simulink model "HEVP0"  (R2026b)
settings: Solver=VariableStepAuto
undefined symbols (not defined in the file): Diff, Eng, Lock, PlntDiffrntlP0Ratio, PlntDriveshftDamp, PlntDriveshftStiff, PlntTransEffTempBpt, PlntTransGearRatioVect, Trans, up
libraries: autolibsharedcoupling x2, autolibsharedtransfixedgear x1, autolibtrqconv x1, autolibpowerinfoutils x1
settings Model: ModifiedByFormat=The MathWorks, Inc.  Creator=The MathWorks, Inc.  LastModifiedBy=The MathWorks, Inc.
settings RTWCC: DLArmComputeVersion=19.05

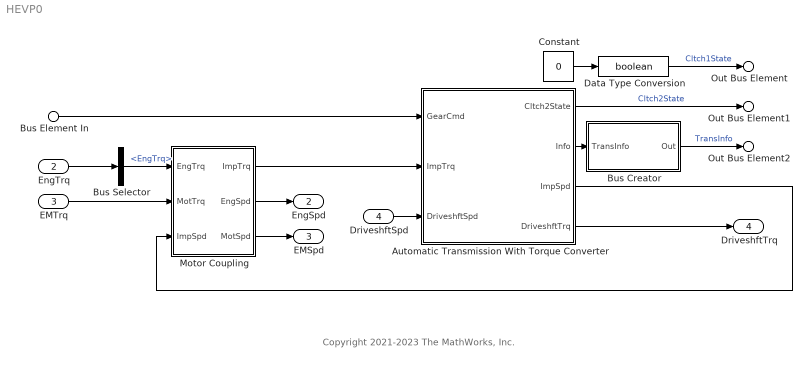
== system HEVP0 ==
  note: Copyright 2021-2023 The MathWorks, Inc.
  Bus Element In : Inport  PortName=Cntrl  Element=Trans.GearCmd
  EngTrq : Inport  Port=2
  EMTrq : Inport  Port=3
  DriveshftSpd : Inport  Port=4
  Automatic Transmission With Torque Converter : Subsystem  VariantControl=1
  Bus Selector : BusSelector  OutputSignals=EngTrq
  Bus Creator : Subsystem
  Constant : Constant  Value=0  SampleTime=-1
  Data Type Conversion : DataTypeConversion  OutDataTypeStr=boolean  SaturateOnIntegerOverflow=off  RndMeth=Floor
  Motor Coupling : Subsystem
  Out Bus Element : Outport  PortName=TransInfo  Element=Cltch1State
  Out Bus Element1 : Outport  PortName=TransInfo  Element=Cltch2State
  Out Bus Element2 : Outport  PortName=TransInfo  Element=Info
  EngSpd : Outport  Port=2  VectorParamsAs1DForOutWhenUnconnected=off  BusOutputAsStruct=on
  EMSpd : Outport  Port=3  VectorParamsAs1DForOutWhenUnconnected=off  BusOutputAsStruct=on
  DriveshftTrq : Outport  Port=4  VectorParamsAs1DForOutWhenUnconnected=off
  wires:
  Automatic Transmission With Torque Converter/4(DriveshftTrq) -> DriveshftTrq/1
  DriveshftSpd/1 -> Automatic Transmission With Torque Converter/3(DriveshftSpd)
  Motor Coupling/2(EngSpd) -> EngSpd/1
  Motor Coupling/3(MotSpd) -> EMSpd/1
  EngTrq/1 -> Bus Selector/1
  EMTrq/1 -> Motor Coupling/2(MotTrq)
  Motor Coupling/1(ImpTrq) -> Automatic Transmission With Torque Converter/2(ImpTrq)
  Bus Element In/1 -> Automatic Transmission With Torque Converter/1(GearCmd)
  Automatic Transmission With Torque Converter/3(ImpSpd) -> Motor Coupling/3(ImpSpd)
  Data Type Conversion/1 -> Out Bus Element/1  "Cltch1State"
  Automatic Transmission With Torque Converter/1(Cltch2State) -> Out Bus Element1/1  "Cltch2State"
  Constant/1 -> Data Type Conversion/1
  Bus Creator/1(Out) -> Out Bus Element2/1  "TransInfo"
  Bus Selector/1 -> Motor Coupling/1(EngTrq)  "<EngTrq>"
  Automatic Transmission With Torque Converter/2(Info) -> Bus Creator/1(TransInfo)

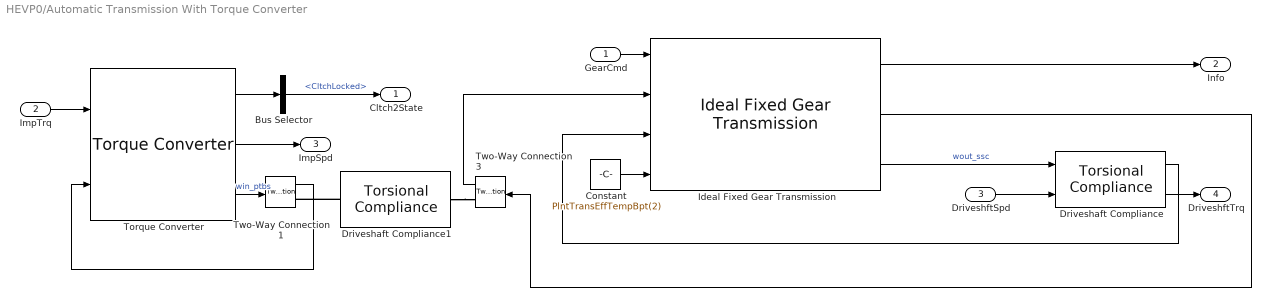
== system HEVP0/Automatic Transmission With Torque Converter ==
  GearCmd : Inport
  ImpTrq : Inport  Port=2
  DriveshftSpd : Inport  Port=3
  Bus Selector : BusSelector  OutputSignals=Cltch.CltchLocked
  Constant : Constant  Value=PlntTransEffTempBpt(2)  SampleTime=-1
  Driveshaft Compliance : autolibsharedcoupling/Torsional Compliance  port_config=Simulink  extInfo=off  k=PlntDriveshftStiff  b=PlntDriveshftDamp  theta_o=PlntDriveshftInitDeflect  domega_o=PlntDriveshftInitVel  omega_c=PlntDriveshftDampCutoffFreq  blkID=0  aMode=1
  Driveshaft Compliance1 : autolibsharedcoupling/Torsional Compliance  port_config=Two-way connection  extInfo=off  k=PlntDriveshftStiff  b=PlntDriveshftDamp  theta_o=PlntDriveshftInitDeflect  domega_o=PlntDriveshftInitVel  omega_c=PlntDriveshftDampCutoffFreq  blkID=0  aMode=1
  Ideal Fixed Gear Transmission : autolibsharedtransfixedgear/Ideal Fixed Gear Transmission  VariantControl=0  TransEffModelPopup=Gear, input torque, input speed, and temperature  gearInterp=Linear point-slope  TrqCnvrtrType=None  G=PlntTransGearNumVect  Trq_bpts=PlntTransEffTrqBpt  omega_bpts=PlntTransEffSpdBpt  Temp_bpts=PlntTransEffTempBpt  N=PlntTransGearRatioVect  Jout=PlntTransInertiaVect  bout=PlntTransDampVect  eta=PlntTransEffVect  eta_tbl=PlntTransEffTbl  G_o=PlntTransInitGear  omega_o=PlntTransInitOutVel  omegaN_o=PlntTransInitNtrlInVel  tau_s=PlntTransShftTimeCnst  phi=[ 0 0.50 0.60 0.70 0.80 0.87 0.92 0.94 0.96 0.97]  psi=[12.2938 12.8588 13.1452 13.6285 14.6163 16.2675 19.3503 22.1046 29.9986 50.00]  zeta=[ 2.2320 1.5462 1.4058 1.2746 1.1528 1.0732 1.0192 0.9983 0.9983 0.9983]  philu=0.96  omegau=0  omegal=0  tauTC=0.1  maxAbsSpd=5e3  aMode=6
  Torque Converter : autolibtrqconv/Torque Converter  TCType=Lock-up  port_config=Simulink  Ji=PlntTrqConvrtrImpInertia  bi=PlntTrqConvrtrImpDamp  Jt=PlntTrqConvrtrTurbInertia  bt=PlntTrqConvrtrTurbDamp  omegai_o=PlntTrqConvrtrImpInitVel  omegat_o=PlntTrqConvrtrTurbInitVel  phi=PlntTrqConvrtrSpdRatioVect  KType=Input speed / sqrt(input torque)  psi=PlntTrqConvrtrCapVect  zeta=PlntTrqConvrtrTrqRatioVect  tauTC=PlntTrqConvrtrTimeCnst  InterpMethod=Linear  Reff=PlntTrqConvrtrCltchRadius  mus=PlntTrqConvrtrCltchStatFric  muk=PlntTrqConvrtrCltchKinFric  ClutchLocked=off  philu=PlntTrqConvrtrCltchLckUpSpdRatio  omegal=PlntTrqConvrtrCltchMinLckUpEngdSpd  omegau=PlntTrqConvrtrCltchMinLckUpDisengdSpd  K_c=PlntTrqConvrtrCltchLckUpForceGain  tauC=PlntTrqConvrtrCltchLckUpTimeCnst  maxAbsSpd=5e3  tau_dl=3000
      settings: AttributesFormatString="Lock-up type:  %<TCType>"
  Two-Way Connection1 : TwoWayConnection
  Two-Way Connection3 : TwoWayConnection
  Cltch2State : Outport  VectorParamsAs1DForOutWhenUnconnected=off
  Info : Outport  Port=2  VectorParamsAs1DForOutWhenUnconnected=off
  ImpSpd : Outport  Port=3  VectorParamsAs1DForOutWhenUnconnected=off
  DriveshftTrq : Outport  Port=4  VectorParamsAs1DForOutWhenUnconnected=off
  wires:
  DriveshftSpd/1 -> Driveshaft Compliance/2
  Torque Converter/3 -> Two-Way Connection1/1  "win_ptbs"
  Two-Way Connection3/1 -> Ideal Fixed Gear Transmission/2
  Torque Converter/2 -> ImpSpd/1
  ImpTrq/1 -> Torque Converter/1
  GearCmd/1 -> Ideal Fixed Gear Transmission/1
  Ideal Fixed Gear Transmission/1 -> Info/1
  Torque Converter/1 -> Bus Selector/1
  Ideal Fixed Gear Transmission/2 -> Two-Way Connection3/1
  Driveshaft Compliance/1 -> Ideal Fixed Gear Transmission/3
  Two-Way Connection1/1 -> Torque Converter/2
  Ideal Fixed Gear Transmission/3 -> Driveshaft Compliance/1  "wout_ssc"
  Bus Selector/1 -> Cltch2State/1  "<CltchLocked>"
  Constant/1 -> Ideal Fixed Gear Transmission/4
  Driveshaft Compliance/2 -> DriveshftTrq/1
  connections:
  Driveshaft Compliance1/RConn1 -- Two-Way Connection3/RConn1
  Driveshaft Compliance1/LConn1 -- Two-Way Connection1/RConn1

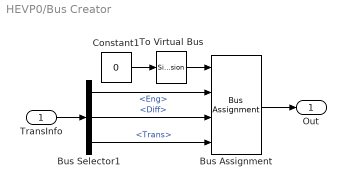
== system HEVP0/Bus Creator ==
  TransInfo : Inport
  Bus Assignment : BusAssignment  AssignedSignals=Eng,Diff,Trans
  Bus Selector1 : BusSelector  OutputSignals=Eng,Diff,Trans
  Constant1 : Constant  Value=0  OutDataTypeStr=Bus: InfoBUS  SampleTime=Inf
  To Virtual Bus : SignalConversion  ConversionOutput=Virtual bus  OverrideOpt=off
  Out : Outport
  wires:
  To Virtual Bus/1 -> Bus Assignment/1
  Constant1/1 -> To Virtual Bus/1
  TransInfo/1 -> Bus Selector1/1
  Bus Selector1/3 -> Bus Assignment/4  "<Trans>"
  Bus Selector1/1 -> Bus Assignment/2  "<Eng>"
  Bus Selector1/2 -> Bus Assignment/3  "<Diff>"
  Bus Assignment/1 -> Out/1

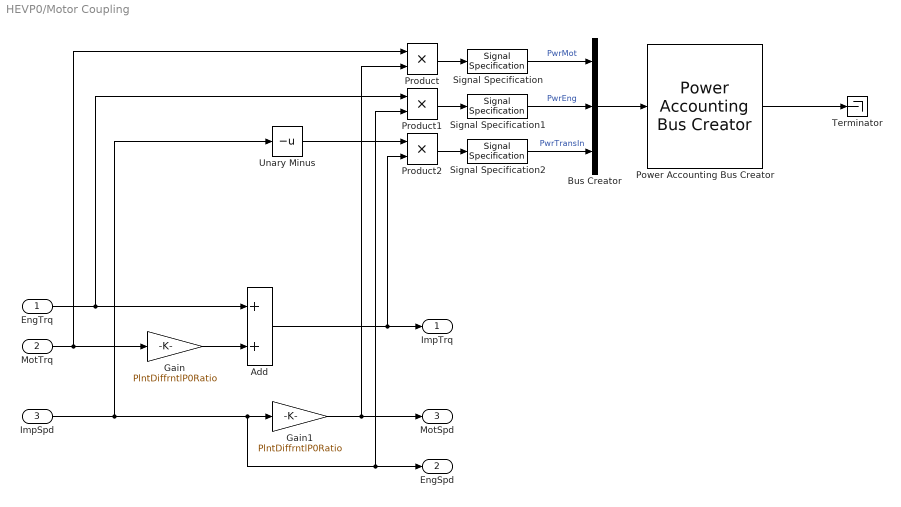
== system HEVP0/Motor Coupling ==
  EngTrq : Inport
  MotTrq : Inport  Port=2
  ImpSpd : Inport  Port=3
  Add : Sum
  Bus Creator : BusCreator  Inputs=3
  Gain : Gain  Gain=PlntDiffrntlP0Ratio
  Gain1 : Gain  Gain=PlntDiffrntlP0Ratio
  Power Accounting Bus Creator : autolibpowerinfoutils/Power Accounting Bus Creator  AssctBlkSelPopup=Parent  RefBlkName='libraryname/blkname'  PwrTrnsfrdCheckBox=on  PwrNotTrnsfrdCheckBox=off  PwrStoredCheckBox=off  aMode=aMode
  Product : Product
  Product1 : Product
  Product2 : Product
  Signal Specification : SignalSpecification  Unit=W
  Signal Specification1 : SignalSpecification  Unit=W
  Signal Specification2 : SignalSpecification  Unit=W
  Terminator : Terminator
  Unary Minus : UnaryMinus
  ImpTrq : Outport  VectorParamsAs1DForOutWhenUnconnected=off
  EngSpd : Outport  Port=2  VectorParamsAs1DForOutWhenUnconnected=off  BusOutputAsStruct=on
  MotSpd : Outport  Port=3  VectorParamsAs1DForOutWhenUnconnected=off  BusOutputAsStruct=on
  wires:
  Unary Minus/1 -> Product2/1
  Product2/1 -> Signal Specification2/1
  Product1/1 -> Signal Specification1/1
  Product/1 -> Signal Specification/1
  Signal Specification1/1 -> Bus Creator/2  "PwrEng"
  Power Accounting Bus Creator/1 -> Terminator/1
  Signal Specification/1 -> Bus Creator/1  "PwrMot"
  Bus Creator/1 -> Power Accounting Bus Creator/1
  Signal Specification2/1 -> Bus Creator/3  "PwrTransIn"
  Gain1/1 -> Product/2, MotSpd/1
  ImpSpd/1 -> Gain1/1, EngSpd/1, Product1/2, Unary Minus/1
  Add/1 -> ImpTrq/1, Product2/2
  EngTrq/1 -> Add/1, Product1/1
  Gain/1 -> Add/2
  MotTrq/1 -> Gain/1, Product/1
